simulink model "untitled"  (R2018a)
settings: Solver=VariableStepAuto  StartTime=0.0  StopTime=10.0  RelTol=1e-3
undefined symbols (not defined in the file): Ka, N
libraries: powerlib x6
settings Model: Creator=enes_  LastModifiedBy=enes_

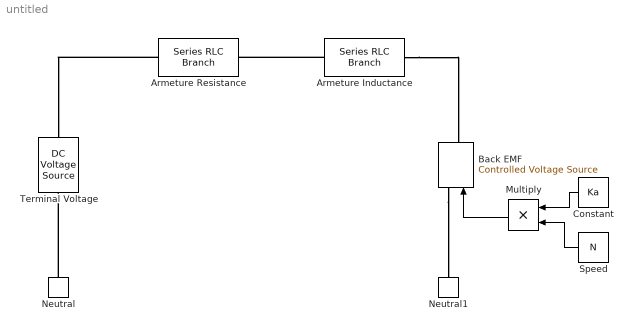
== system untitled ==
  Armeture Inductance : powerlib/Elements/Series RLC Branch  LConnTagsString=__new0  RConnTagsString=__new0  BranchType=L  Resistance=1  Inductance=1e-3  SetiL0=off  InitialCurrent=0  Capacitance=1e-6  Setx0=off  InitialVoltage=0  Measurements=None
  "Armeture Resistance " : powerlib/Elements/Series RLC Branch  LConnTagsString=__new0  RConnTagsString=__new0  BranchType=R  Resistance=1  Inductance=1e-3  SetiL0=off  InitialCurrent=0  Capacitance=1e-6  Setx0=off  InitialVoltage=0  Measurements=None
  Back EMF : powerlib/Electrical Sources/Controlled Voltage Source  Initialize=on  Source_Type=AC  Amplitude=0  Phase=0  Frequency=0  Measurements=None
  Constant : Constant  Value=Ka
  Multiply : Product
  Neutral : powerlib/Elements/Neutral  LConnTagsString=a  NodeNumber=10
      settings: SourceProductName=Simscape Power Systems  SourceProductBaseCode=PS
  Neutral1 : powerlib/Elements/Neutral  LConnTagsString=a  NodeNumber=10
      settings: SourceProductName=Simscape Power Systems  SourceProductBaseCode=PS
  "Speed " : Constant  Value=N
  Terminal Voltage : powerlib/Electrical Sources/DC Voltage Source  Amplitude=100  Measurements=None
  wires:
  Multiply/1 -> Back EMF/1
  "Speed "/1 -> Multiply/2
  Constant/1 -> Multiply/1
  connections:
  "Armeture Resistance "/LConn1 -- Terminal Voltage/RConn1
  Armeture Inductance/RConn1 -- Back EMF/RConn1
  Neutral/LConn1 -- Terminal Voltage/LConn1
  Armeture Inductance/LConn1 -- "Armeture Resistance "/RConn1
  Back EMF/LConn1 -- Neutral1/LConn1
